simulink model "controlScheme_DS"  (R2019b)
settings: Solver=FixedStepDiscrete  StartTime=0.0  StopTime=Inf  FixedStep=1/30  RelTol=1e-3
InitFcn:
  | %tb = twinbeam('147.32.86.177', 30000);
  | %gen = generator('147.32.86.177', 30001);
  | %img = tb.get();
  | %f = figure(25)
  | %imshow(img);
  | %[x_0, y_0] = ginput(1);
  | 
  | x_0 = 200;
  | y_0 = 200;
  | 
  | %delete(tb)
  | %delete(gen)
  | %pause(4)
  | %close(f)
model workspace (MAT data in the model file):
  NumberOfBeads = Simulink.Parameter
  NumberOfBeads.Value = 1
  NumberOfBeads.DataType = 'auto'
  NumberOfBeads.Dimensions = [1 1]
undefined symbols (not defined in the file): DiscIntNeverNeededParam, H, Joystick, Standard_Devices, TCP_Protocol
libraries: sldrtlib x7, simulink x1
settings Model: SimulationMode=accelerator  EnablePacing=on  ParameterArgumentNames=NumberOfBeads  OrderedModelArguments=off  Creator=marti  LastModifiedBy=marti
settings SolverCC: MinimalZcImpactIntegration=on
settings DebuggingCC: ReadBeforeWriteMsg=DisableAll  WriteAfterWriteMsg=DisableAll  WriteAfterReadMsg=DisableAll  MultiTaskDSMMsg=none
settings ModelReferenceCC: UpdateModelReferenceTargets=IfOutOfDate
settings SFSimCC: SFSimEcho=off
settings RTWCC: Description=Simulink Desktop Real-Time  SystemTargetFile=sldrt.tlc  TemplateMakefile=sldrt.tmf  RTWCompilerOptimization=on
settings CodeAppCC: MaxIdLength=95
settings SimulinkDesktopRealTimeCC: TargetPreCompLibLocation=C:\Program Files\MATLAB\R2020a\toolbox\sldrt\lib\win64

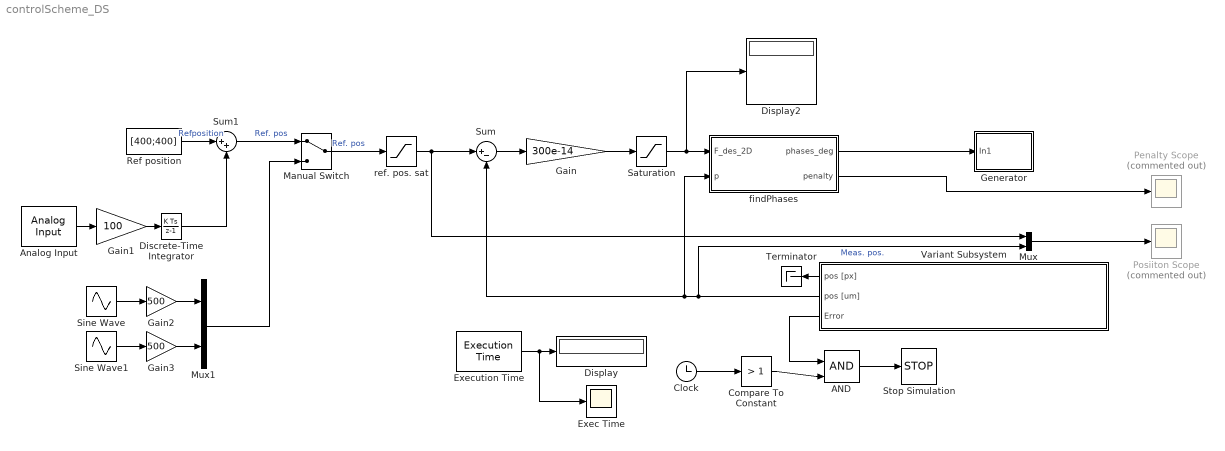
== system controlScheme_DS ==
  AND : Logic  IconShape=distinctive  AllPortsSameDT=off  OutDataTypeStr=boolean
  Analog Input : sldrtlib/Analog Input  SampleTime=0.1  MaxMissedTicks=10  ShowMissedTicks=off  YieldWhenWaiting=off  DrvName=Standard_Devices/Joystick  DrvAddress=1  DrvOptions=zeros(1,0)  Channels=[1:2]  RangeMode=1  VoltRange=1  DataType=1
      settings: AttributesFormatString=Joystick [1]
  Clock : Clock
  Compare To Constant : simulink/Logic and Bit Operations/Compare To Constant  relop=>  const=1  OutDataTypeStr=boolean
  Discrete-Time Integrator : DiscreteIntegrator  gainval=1  SampleTime=-1  ICPrevOutput=DiscIntNeverNeededParam  ICPrevScaledInput=DiscIntNeverNeededParam
  Display : Display
  Display2 : Display
  Exec Time : Scope
  Execution Time : sldrtlib/Target Profiling/Execution Time  ShowTaskTimes=off
      settings: SourceProductBaseCode=WT
  Gain : Gain  Gain=300e-14
  Gain1 : Gain  Gain=100
  Gain2 : Gain  Gain=500
  Gain3 : Gain  Gain=500
  Generator : Subsystem
  Manual Switch : ManualSwitch
  Mux : Mux  Inputs=2
  Mux1 : Mux  Inputs=2
  Penalty Scope : Scope  Commented=on
  Posiiton Scope : Scope  Commented=on
  Ref position : Constant  Value=[400;400]
  Saturation : Saturate  UpperLimit=20e-11  LowerLimit=-20e-11
  Sine Wave : Sin  Frequency=2*pi/40  SampleTime=0
  Sine Wave1 : Sin  Frequency=2*pi/20  Phase=-pi  SampleTime=0
  Stop Simulation : Stop
  Sum : Sum  Inputs=|+-
  Sum1 : Sum  Inputs=|++
  Terminator : Terminator
  Variant Subsystem : Subsystem  Variant=on
  findPhases : MATLAB Function  TreatAsAtomicUnit=on
  ref. pos. sat : Saturate  UpperLimit=600  LowerLimit=-600
  wires:
  Manual Switch/1 -> ref. pos. sat/1  "Ref. pos"
  Sum/1 -> Gain/1
  Gain/1 -> Saturation/1
  Saturation/1 -> findPhases/1(F_des_2D), Display2/1
  Variant Subsystem/2(pos [um]) -> Mux/2, findPhases/2(p), Sum/2  "Meas. pos."
  Execution Time/1 -> Exec Time/1, Display/1
  findPhases/1(phases_deg) -> Generator/1(In1)
  findPhases/2(penalty) -> Penalty Scope/1
  AND/1 -> Stop Simulation/1
  Clock/1 -> Compare To Constant/1
  Compare To Constant/1 -> AND/2
  Variant Subsystem/3(Error) -> AND/1
  Mux/1 -> Posiiton Scope/1
  Analog Input/1 -> Gain1/1
  Ref position/1 -> Sum1/1  "Refposition"
  Discrete-Time Integrator/1 -> Sum1/2
  Gain1/1 -> Discrete-Time Integrator/1
  Sum1/1 -> Manual Switch/1  "Ref. pos"
  Sine Wave/1 -> Gain2/1
  Sine Wave1/1 -> Gain3/1
  Gain2/1 -> Mux1/1
  Gain3/1 -> Mux1/2
  Mux1/1 -> Manual Switch/2
  Variant Subsystem/1(pos [px]) -> Terminator/1
  ref. pos. sat/1 -> Sum/1, Mux/1

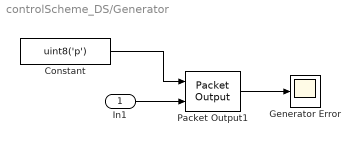
== system controlScheme_DS/Generator ==
  In1 : Inport
  Constant : Constant  Value=uint8('p')
  Generator Error : Scope
  Packet Output1 : sldrtlib/Packet Output  SampleTime=1/30  MaxMissedTicks=20  ShowMissedTicks=off  YieldWhenWaiting=off  DrvName=Standard_Devices/TCP_Protocol  DrvAddress=30001  DrvOptions=[0 30001 49 52 55 46 51 50 46 56 54 46 49 55 55 0 0 0 0 0 0 0 0 0 0 0 0 0 0 0 0 0 0 0 0 0 0 0 0 0 0 0 0 0 0 0 0 0 0 0 0 0 0 0 0 0 0 0 0 0 0 0 0 0 0 0 0 0 0 0 0 0 0 0 0 0 0 0 0 0 0 0 0 0 0 0 0 0 0 0 0 0 0 0 0 0 0 0 0 0 0 0 0 0 0 0 0 0 0 0 0 0 0 0 0 0 0 0 0 0 0 0 0 0 0 0 0 0 0 0 0 0 0 0 0 0 0 0 0 0 0 0 0 0 0 0 0 0 0 0 0 0 0 0 0 0 0 0 0 0 0 0 0 0 0 0 0 0 0 0 0 0 0 0 0 0 0 0 0 0 0 0 0 0 0 0 0 0 0 0 0 0 0 0 0 0 0 0 0 0 0 0 0 0 0 0 0 0 0 0 0 0 0 0 0 0 0 0 0 0 0 0 0 0 0 0 0 0 0 0 0 0 0 0 0 0 0 0 0 0 0 0 0 0 0 0 0 0 0 0 0 0 0 0 0 0]  PacketSize=56*2+1  DataTypes={'uint8', '56*uint16'}  ShowReady=off  ShowError=on  PacketID=1  ByteOrder=1  InitialValue=[]  FinalValue=[]
      settings: AttributesFormatString=TCP Protocol [30001]
  wires:
  In1/1 -> Packet Output1/2
  Packet Output1/1 -> Generator Error/1
  Constant/1 -> Packet Output1/1

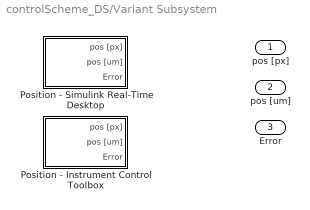
== system controlScheme_DS/Variant Subsystem ==
  Position - Instrument Control Toolbox : Subsystem  VariantControl=instrumentControlToolbox==true
  Position - Simulink Real-Time Desktop : Subsystem  VariantControl=(default)
  pos [px] : Outport
  pos [um] : Outport  Port=2
  Error : Outport  Port=3

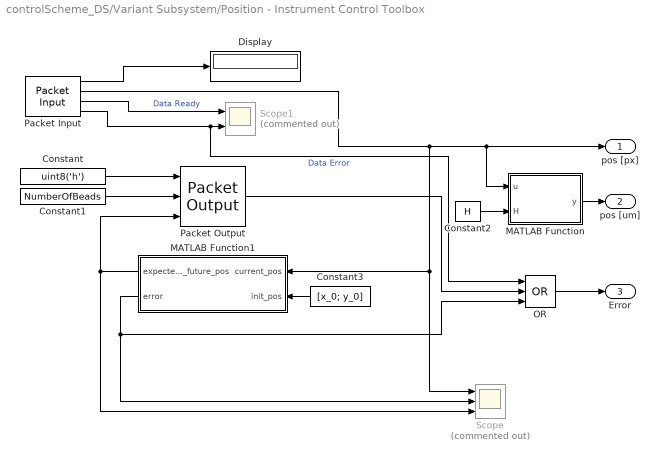
== system controlScheme_DS/Variant Subsystem/Position - Instrument Control Toolbox ==
  Constant : Constant  Value=uint8('h')  OutDataTypeStr=uint8  SampleTime=-1
  Constant1 : Constant  Value=NumberOfBeads  OutDataTypeStr=uint32  SampleTime=-1
  Constant2 : Constant  Value=H
  Constant3 : Constant  Value=[x_0; y_0]
  Display : Display
      settings: Format=decimal (Stored Integer)
  MATLAB Function : MATLAB Function  TreatAsAtomicUnit=on
  MATLAB Function1 : MATLAB Function  TreatAsAtomicUnit=on
  OR : Logic  Operator=OR  Inputs=3  IconShape=distinctive  AllPortsSameDT=off  OutDataTypeStr=boolean
  Packet Input : sldrtlib/Packet Input  SampleTime=1/30  MaxMissedTicks=20  ShowMissedTicks=off  YieldWhenWaiting=off  DrvName=Standard_Devices/TCP_Protocol  DrvAddress=30000  DrvOptions=[0 30000 49 52 55 46 51 50 46 56 54 46 49 55 55 0 0 0 0 0 0 0 0 0 0 0 0 0 0 0 0 0 0 0 0 0 0 0 0 0 0 0 0 0 0 0 0 0 0 0 0 0 0 0 0 0 0 0 0 0 0 0 0 0 0 0 0 0 0 0 0 0 0 0 0 0 0 0 0 0 0 0 0 0 0 0 0 0 0 0 0 0 0 0 0 0 0 0 0 0 0 0 0 0 0 0 0 0 0 0 0 0 0 0 0 0 0 0 0 0 0 0 0 0 0 0 0 0 0 0 0 0 0 0 0 0 0 0 0 0 0 0 0 0 0 0 0 0 0 0 0 0 0 0 0 0 0 0 0 0 0 0 0 0 0 0 0 0 0 0 0 0 0 0 0 0 0 0 0 0 0 0 0 0 0 0 0 0 0 0 0 0 0 0 0 0 0 0 0 0 0 0 0 0 0 0 0 0 0 0 0 0 0 0 0 0 0 0 0 0 0 0 0 0 0 0 0 0 0 0 0 0 0 0 0 0 0 0 0 0 0 0 0 0 0 0 0 0 0 0 0 0 0 0 0 0]  PacketSize=4+4  DataTypes={'uint32', '2*uint16'}  ShowReady=on  ShowError=on  PacketID=1  ByteOrder=1  ShowTimestamp=off
      settings: AttributesFormatString=TCP Protocol [30000]
  Packet Output : sldrtlib/Packet Output  SampleTime=1/30  MaxMissedTicks=20  ShowMissedTicks=off  YieldWhenWaiting=off  DrvName=Standard_Devices/TCP_Protocol  DrvAddress=30000  DrvOptions=[0 30000 49 52 55 46 51 50 46 56 54 46 49 55 55 0 0 0 0 0 0 0 0 0 0 0 0 0 0 0 0 0 0 0 0 0 0 0 0 0 0 0 0 0 0 0 0 0 0 0 0 0 0 0 0 0 0 0 0 0 0 0 0 0 0 0 0 0 0 0 0 0 0 0 0 0 0 0 0 0 0 0 0 0 0 0 0 0 0 0 0 0 0 0 0 0 0 0 0 0 0 0 0 0 0 0 0 0 0 0 0 0 0 0 0 0 0 0 0 0 0 0 0 0 0 0 0 0 0 0 0 0 0 0 0 0 0 0 0 0 0 0 0 0 0 0 0 0 0 0 0 0 0 0 0 0 0 0 0 0 0 0 0 0 0 0 0 0 0 0 0 0 0 0 0 0 0 0 0 0 0 0 0 0 0 0 0 0 0 0 0 0 0 0 0 0 0 0 0 0 0 0 0 0 0 0 0 0 0 0 0 0 0 0 0 0 0 0 0 0 0 0 0 0 0 0 0 0 0 0 0 0 0 0 0 0 0 0 0 0 0 0 0 0 0 0 0 0 0 0 0 0 0 0 0 0]  PacketSize=1+4+4  DataTypes={'uint8', 'uint32', '2*uint16'}  ShowReady=off  ShowError=on  PacketID=1  ByteOrder=1  InitialValue=[]  FinalValue=[]
      settings: AttributesFormatString=TCP Protocol [30000]
  Scope : Scope  Commented=on  NumInputPorts=3
  Scope1 : Scope  Commented=on  NumInputPorts=2
  pos [px] : Outport
  pos [um] : Outport  Port=2  Unit=um
  Error : Outport  Port=3
  wires:
  Constant1/1 -> Packet Output/2
  Packet Input/4 -> OR/1, Scope1/2  "Data Error"
  Packet Input/2 -> MATLAB Function/1(u), pos [px]/1, MATLAB Function1/1(current_pos), Scope/1
  Packet Input/1 -> Display/1
  Packet Input/3 -> Scope1/1  "Data Ready"
  Constant/1 -> Packet Output/1
  Constant2/1 -> MATLAB Function/2(H)
  MATLAB Function/1(y) -> pos [um]/1
  OR/1 -> Error/1
  Packet Output/1 -> OR/2
  MATLAB Function1/1(expected_future_pos) -> Scope/3, Packet Output/3
  MATLAB Function1/2(error) -> Scope/2, OR/3
  Constant3/1 -> MATLAB Function1/2(init_pos)

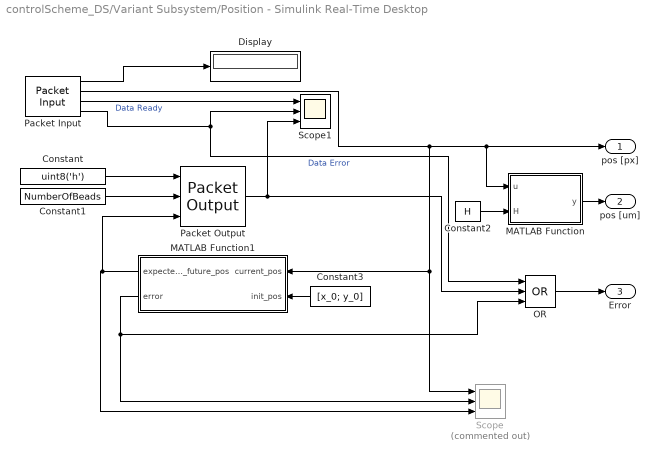
== system controlScheme_DS/Variant Subsystem/Position - Simulink Real-Time Desktop ==
  Constant : Constant  Value=uint8('h')  OutDataTypeStr=uint8  SampleTime=-1
  Constant1 : Constant  Value=NumberOfBeads  OutDataTypeStr=uint32  SampleTime=-1
  Constant2 : Constant  Value=H
  Constant3 : Constant  Value=[x_0; y_0]
  Display : Display
      settings: Format=decimal (Stored Integer)
  MATLAB Function : MATLAB Function  TreatAsAtomicUnit=on
  MATLAB Function1 : MATLAB Function  TreatAsAtomicUnit=on
  OR : Logic  Operator=OR  Inputs=3  IconShape=distinctive  AllPortsSameDT=off  OutDataTypeStr=boolean
  Packet Input : sldrtlib/Packet Input  SampleTime=1/30  MaxMissedTicks=20  ShowMissedTicks=off  YieldWhenWaiting=off  DrvName=Standard_Devices/TCP_Protocol  DrvAddress=30002  DrvOptions=[0 30000 49 52 55 46 51 50 46 56 54 46 49 55 55 0 0 0 0 0 0 0 0 0 0 0 0 0 0 0 0 0 0 0 0 0 0 0 0 0 0 0 0 0 0 0 0 0 0 0 0 0 0 0 0 0 0 0 0 0 0 0 0 0 0 0 0 0 0 0 0 0 0 0 0 0 0 0 0 0 0 0 0 0 0 0 0 0 0 0 0 0 0 0 0 0 0 0 0 0 0 0 0 0 0 0 0 0 0 0 0 0 0 0 0 0 0 0 0 0 0 0 0 0 0 0 0 0 0 0 0 0 0 0 0 0 0 0 0 0 0 0 0 0 0 0 0 0 0 0 0 0 0 0 0 0 0 0 0 0 0 0 0 0 0 0 0 0 0 0 0 0 0 0 0 0 0 0 0 0 0 0 0 0 0 0 0 0 0 0 0 0 0 0 0 0 0 0 0 0 0 0 0 0 0 0 0 0 0 0 0 0 0 0 0 0 0 0 0 0 0 0 0 0 0 0 0 0 0 0 0 0 0 0 0 0 0 0 0 0 0 0 0 0 0 0 0 0 0 0 0 0 0 0 0 0]  PacketSize=4+4  DataTypes={'uint32', '2*uint16'}  ShowReady=on  ShowError=on  PacketID=1  ByteOrder=1  ShowTimestamp=off
      settings: AttributesFormatString=TCP Protocol [30002]
  Packet Output : sldrtlib/Packet Output  SampleTime=1/30  MaxMissedTicks=20  ShowMissedTicks=off  YieldWhenWaiting=off  DrvName=Standard_Devices/TCP_Protocol  DrvAddress=30002  DrvOptions=[0 30000 49 52 55 46 51 50 46 56 54 46 49 55 55 0 0 0 0 0 0 0 0 0 0 0 0 0 0 0 0 0 0 0 0 0 0 0 0 0 0 0 0 0 0 0 0 0 0 0 0 0 0 0 0 0 0 0 0 0 0 0 0 0 0 0 0 0 0 0 0 0 0 0 0 0 0 0 0 0 0 0 0 0 0 0 0 0 0 0 0 0 0 0 0 0 0 0 0 0 0 0 0 0 0 0 0 0 0 0 0 0 0 0 0 0 0 0 0 0 0 0 0 0 0 0 0 0 0 0 0 0 0 0 0 0 0 0 0 0 0 0 0 0 0 0 0 0 0 0 0 0 0 0 0 0 0 0 0 0 0 0 0 0 0 0 0 0 0 0 0 0 0 0 0 0 0 0 0 0 0 0 0 0 0 0 0 0 0 0 0 0 0 0 0 0 0 0 0 0 0 0 0 0 0 0 0 0 0 0 0 0 0 0 0 0 0 0 0 0 0 0 0 0 0 0 0 0 0 0 0 0 0 0 0 0 0 0 0 0 0 0 0 0 0 0 0 0 0 0 0 0 0 0 0 0]  PacketSize=1+4+4  DataTypes={'uint8', 'uint32', '2*uint16'}  ShowReady=off  ShowError=on  PacketID=1  ByteOrder=1  InitialValue=[]  FinalValue=[]
      settings: AttributesFormatString=TCP Protocol [30002]
  Scope : Scope  Commented=on  NumInputPorts=3
  Scope1 : Scope  NumInputPorts=3
  pos [px] : Outport
  pos [um] : Outport  Port=2  Unit=um
  Error : Outport  Port=3
  wires:
  Packet Input/4 -> OR/1, Scope1/2  "Data Error"
  Packet Input/2 -> MATLAB Function/1(u), pos [px]/1, MATLAB Function1/1(current_pos), Scope/1
  Packet Input/1 -> Display/1
  Packet Input/3 -> Scope1/1  "Data Ready"
  Constant/1 -> Packet Output/1
  Constant2/1 -> MATLAB Function/2(H)
  MATLAB Function/1(y) -> pos [um]/1
  OR/1 -> Error/1
  Packet Output/1 -> OR/2, Scope1/3
  MATLAB Function1/1(expected_future_pos) -> Packet Output/3, Scope/3
  MATLAB Function1/2(error) -> OR/3, Scope/2
  Constant3/1 -> MATLAB Function1/2(init_pos)
  Constant1/1 -> Packet Output/2

== matlab function controlScheme_DS/findPhases ==
  data: F_des_2D input; p input; phases_deg output; penalty output
function [phases_deg, penalty] = fcn(F_des_2D, p)
ParticleRadisu = 25e-6;
ParticleDensity = 1.05e3;
MediumDensity = 0.998e3;
g = 9.81373; % m/s^2
F_z = -4/3*pi*ParticleRadisu^3*(MediumDensity-ParticleDensity)*g;
F_des = [0;0;F_z];
p_z = 130e-6;
position = [0;0;p_z];

F_des(1:2) = F_des_2D;
position(1:2) = p*1e-6;
[phases_rad, penalty] = findPhasesFoGivenF(position, F_des);
phases_deg = rad2deg(phases_rad);
phases_deg = round(mod(phases_deg, 360));

== matlab function controlScheme_DS/Variant Subsystem/Position - Simulink Real-Time Desktop/MATLAB Function ==
  data: u input; y output; H input
function y = fcn(u, H)
tmp = H*[double(u(2));double(u(1));1];
y = [tmp(1)/tmp(3); tmp(2)/tmp(3)];

== matlab function controlScheme_DS/Variant Subsystem/Position - Simulink Real-Time Desktop/MATLAB Function1 ==
  data: current_pos input; expected_future_pos output; init_pos input; error output
function [expected_future_pos, error] = fcn(current_pos, init_pos)

persistent errr_count old_pos;
if isempty(errr_count)
  errr_count = 0;
  old_pos = uint16(init_pos);
end

error = false;

if (old_pos(1)-current_pos(1))^2 + (old_pos(2)-current_pos(2))^2 < 50^2
    errr_count = 0;
    expected_future_pos = current_pos;
    old_pos = current_pos;
else
    errr_count = errr_count + 1;
    expected_future_pos = old_pos;
    
    if errr_count > 10
        error = true;
    end
end

== matlab function controlScheme_DS/Variant Subsystem/Position - Instrument Control Toolbox/MATLAB Function ==
  data: u input; y output; H input
function y = fcn(u, H)
tmp = H*[double(u(2));double(u(1));1];
y = [tmp(1)/tmp(3); tmp(2)/tmp(3)];

== matlab function controlScheme_DS/Variant Subsystem/Position - Instrument Control Toolbox/MATLAB Function1 ==
  data: current_pos input; expected_future_pos output; init_pos input; error output
function [expected_future_pos, error] = fcn(current_pos, init_pos)

persistent errr_count old_pos;
if isempty(errr_count)
  errr_count = 0;
  old_pos = uint16(init_pos);
end

error = false;

if (old_pos(1)-current_pos(1))^2 + (old_pos(2)-current_pos(2))^2 < 50^2
    errr_count = 0;
    expected_future_pos = current_pos;
    old_pos = current_pos;
else
    errr_count = errr_count + 1;
    expected_future_pos = old_pos;
    
    if errr_count > 10
        error = true;
    end
end
